simulink model "isitsame"  (R2014b)
settings: Solver=ode45  StartTime=0.0  StopTime=100.0  RelTol=1e-3
values from neighbouring files (symbols this model uses):
  m0 = (I1*I2*I3*I4)/(Rt1*Rt2*Rt3*Cs)    (= 1)    [vars.m]
  m1 = ((I2*I3*I4)/(Rt2*Rt3*Cs))+(((Rt3*I4+Rt2*I1*I3*(I2+I4))/(Rt1*Rt2*Rt3*Cs)))    (= 4)    [vars.m]
  m2 = (((I1+I3)*(I2*Rt2+I4*(Rt2+Rt3)))/(Rt2*Rt3*Cs))+((I1*I3*(Rt2+Rt3))/(Rt1*Rt3*Cs))    (= 8)    [vars.m]
  m3 = (((I1+I3)*(Rt2+Rt3))/(Rt3*Cs))+((I1*I2*I4)/(Rt1*Rt2*Rt3))+((I1*I2*I3)/(Rt1*Rt2*Rt3))-((I1*I3*Rt2)/(Rt1*Rt3*Cs))    (= 5)    [vars.m]
  m4 = ((2*I1*I2+I2*I3+I2*I4)/(Rt2*Rt3))+((I1*(I3+I4)*(Rt2+Rt3))/(Rt1*Rt2*Rt3))-((Rt2*(I1+I3))/(Rt3*Cs))    (= 6)    [vars.m]
  m5 = (((Rt3+Rt2)*(2*I1+I3+I4))/(Rt3*Rt2))+I2    (= 9)    [vars.m]
  m6 = 1    [vars.m]
  m7 = (2*pi*fi)/(Pn*m*Rx)    (= 6.28318530718)    [vars.m]
settings Model: Creator=Jacek  LastModifiedBy=Jacek

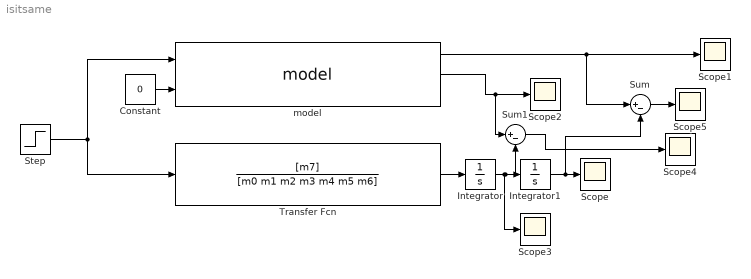
== system isitsame ==
  Constant : Constant  Value=0
  Integrator : Integrator
  Integrator1 : Integrator
  Scope{,1..5} (6 alike) : Scope
      Scope2 settings: SaveName=ScopeData2
      Scope3 settings: SaveName=ScopeData3
      Scope4 settings: SaveName=ScopeData4
      Scope5 settings: SaveName=ScopeData5
  Step : Step  SampleTime=0
  Sum : Sum  Inputs=|+-
  Sum1 : Sum  Inputs=|+-
  Transfer Fcn : TransferFcn  Numerator=[m7]  Denominator=[m0 m1 m2 m3 m4 m5 m6]
  model : S-Function  FunctionName=model  EnableBusSupport=off
      mask Display: port_label('input',1,'Ein.'); port_label('input',2,'Fin.'); port_label('output',1,'Pout.'); port_label('output',2,'Vout.'); port_label('output',3,'DEBUG')
  wires:
  Constant/1 -> model/2
  Step/1 -> Transfer Fcn/1, model/1
  Transfer Fcn/1 -> Integrator/1
  Integrator/1 -> Scope3/1, Sum1/2, Integrator1/1
  Integrator1/1 -> Sum/2, Scope/1
  model/2 -> Sum1/1, Scope2/1
  model/1 -> Sum/1, Scope1/1
  Sum/1 -> Scope5/1
  Sum1/1 -> Scope4/1
